simulink model "sample"  (R2018b)
settings: Solver=FixedStepDiscrete  StartTime=0.0  StopTime=10.0  RelTol=1e-3
libraries: simulink x2
settings Model: Creator=a_miyazaki  LastModifiedBy=a_miyazaki

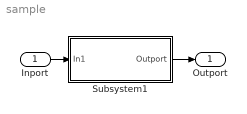
== system sample ==
  Inport : Inport
  Subsystem1 : Subsystem
  Outport : Outport
  wires:
  Inport/1 -> Subsystem1/1(In1)
  Subsystem1/1(Outport) -> Outport/1

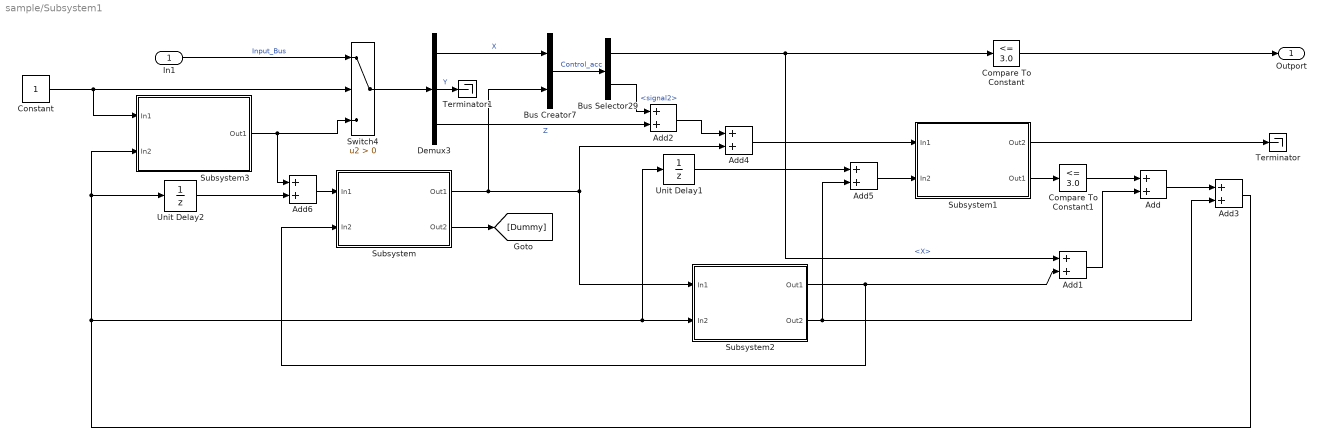
== system sample/Subsystem1 ==
  In1 : Inport
  Add{,1..6} (7 alike) : Sum
  Bus Creator7 : BusCreator  Inputs=2
  Bus Selector29 : BusSelector  OutputSignals=X,signal2
  Compare To Constant : simulink/Logic and Bit Operations/Compare To Constant  relop=<=  const=3.0  OutDataTypeStr=boolean
  Compare To Constant1 : simulink/Logic and Bit Operations/Compare To Constant  relop=<=  const=3.0  OutDataTypeStr=boolean
  Constant : Constant  SampleTime=-1
  Demux3 : Demux  Outputs=3
  Subsystem : Subsystem
  Subsystem1 : Subsystem
  Subsystem2 : Subsystem
  Subsystem3 : Subsystem
  Switch4 : Switch  Criteria=u2 > Threshold
  Terminator : Terminator
  Terminator1 : Terminator
  Unit Delay1 : UnitDelay  SampleTime=-1
  Unit Delay2 : UnitDelay  SampleTime=-1
  Outport : Outport
  wires:
  Subsystem2/2(Out2) -> Add5/2, Add3/2
  Subsystem1/2(Out1) -> Compare To Constant1/1
  Add1/1 -> Add/2
  In1/1 -> Switch4/1  "Input_Bus"
  Switch4/1 -> Demux3/1
  Demux3/1 -> Bus Creator7/1  "X"
  Bus Creator7/1 -> Bus Selector29/1  "Control_acc"
  Bus Selector29/1 -> Compare To Constant/1, Add1/1  "<X>"
  Demux3/3 -> Add2/2  "Z"
  Bus Selector29/2 -> Add2/1  "<signal2>"
  Add2/1 -> Add4/1
  Subsystem/1(Out1) -> Subsystem2/1(In1), Add4/2, Bus Creator7/2
  Demux3/2 -> Terminator1/1  "Y"
  Add4/1 -> Subsystem1/1(In1)
  Add/1 -> Add3/1
  Subsystem3/1(Out1) -> Add6/1, Switch4/3
  Constant/1 -> Subsystem3/1(In1), Switch4/2
  Subsystem2/1(Out1) -> Subsystem/2(In2), Add1/2
  Add3/1 -> Unit Delay1/1, Subsystem2/2(In2), Subsystem3/2(In2), Unit Delay2/1
  Subsystem1/1(Out2) -> Terminator/1
  Subsystem/2(Out2) -> [Dummy]
  Compare To Constant/1 -> Outport/1
  Compare To Constant1/1 -> Add/1
  Add5/1 -> Subsystem1/2(In2)
  Add6/1 -> Subsystem/1(In1)
  Unit Delay1/1 -> Add5/1
  Unit Delay2/1 -> Add6/2

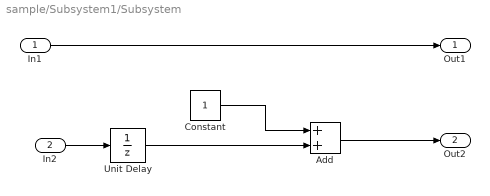
== system sample/Subsystem1/Subsystem ==
  In1 : Inport
  In2 : Inport  Port=2
  Add : Sum
  Constant : Constant  SampleTime=-1
  Unit Delay : UnitDelay  SampleTime=-1
  Out1 : Outport
  Out2 : Outport  Port=2
  wires:
  In1/1 -> Out1/1
  Constant/1 -> Add/1
  Add/1 -> Out2/1
  In2/1 -> Unit Delay/1
  Unit Delay/1 -> Add/2

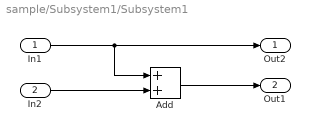
== system sample/Subsystem1/Subsystem1 ==
  In1 : Inport
  In2 : Inport  Port=2
  Add : Sum
  Out2 : Outport
  Out1 : Outport  Port=2
  wires:
  In1/1 -> Add/1, Out2/1
  In2/1 -> Add/2
  Add/1 -> Out1/1

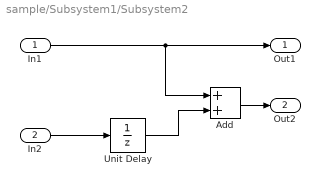
== system sample/Subsystem1/Subsystem2 ==
  In1 : Inport
  In2 : Inport  Port=2
  Add : Sum
  Unit Delay : UnitDelay  SampleTime=-1
  Out1 : Outport
  Out2 : Outport  Port=2
  wires:
  In1/1 -> Add/1, Out1/1
  Add/1 -> Out2/1
  In2/1 -> Unit Delay/1
  Unit Delay/1 -> Add/2

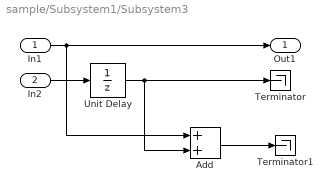
== system sample/Subsystem1/Subsystem3 ==
  In1 : Inport
  In2 : Inport  Port=2
  Add : Sum
  Terminator : Terminator
  Terminator1 : Terminator
  Unit Delay : UnitDelay  SampleTime=-1
  Out1 : Outport
  wires:
  In1/1 -> Add/1, Out1/1
  In2/1 -> Unit Delay/1
  Unit Delay/1 -> Add/2, Terminator/1
  Add/1 -> Terminator1/1
